simulink model "Single_area_lfc_pid"  (R2025a)
settings: Solver=ode4  StartTime=0.0  StopTime=50.0  RelTol=1e-3
settings Model: Creator=sabreen  LastModifiedBy=sabreen

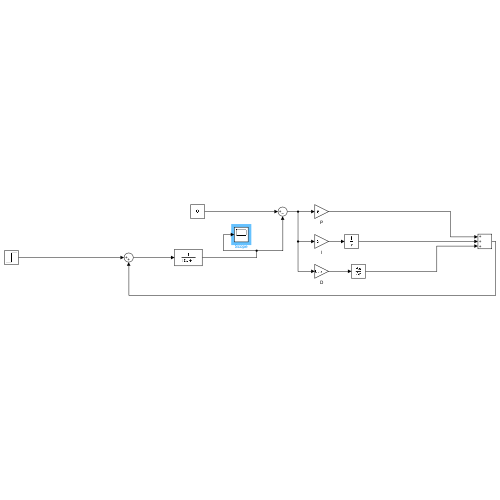
[thumbnail: Simulink's stored preview of the top-level diagram]
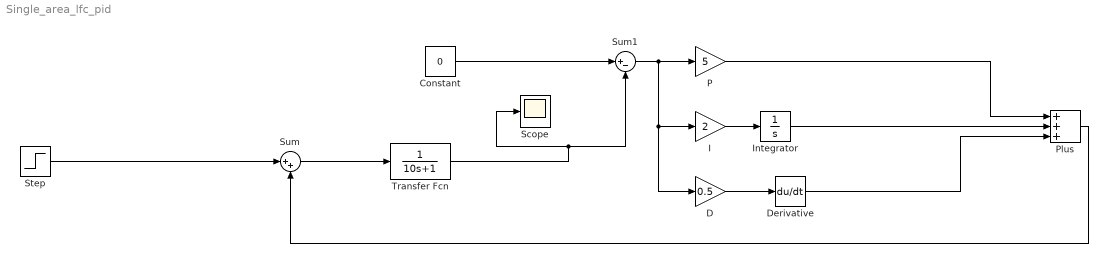
== system Single_area_lfc_pid ==
  Constant : Constant  Value=0
  D : Gain  Gain=0.5
  Derivative : Derivative
  I : Gain  Gain=2
  Integrator : Integrator
  P : Gain  Gain=5
  Plus : Sum  Inputs=+++
  Scope : Scope
      settings: ActiveDisplayYMinimum=-0.00020324478402603376  ActiveDisplayYMaximum=0.0011544135578532868
  Step : Step  Time=0  After=0.01  SampleTime=0
  Sum : Sum  Inputs=|++
  Sum1 : Sum  Inputs=|+-
  Transfer Fcn : TransferFcn  Denominator=[10 1]
  wires:
  Transfer Fcn/1 -> Sum1/2, Scope/1
  Step/1 -> Sum/1
  Sum/1 -> Transfer Fcn/1
  Constant/1 -> Sum1/1
  Sum1/1 -> D/1, I/1, P/1
  I/1 -> Integrator/1
  D/1 -> Derivative/1
  P/1 -> Plus/1
  Integrator/1 -> Plus/2
  Derivative/1 -> Plus/3
  Plus/1 -> Sum/2
